simulink library "Index2DbTableBtc"  (R2022b)
settings: Solver=VariableStepAuto  StartTime=0.0  StopTime=10.0  RelTol=1e-3
undefined symbols (not defined in the file or in its folder): Config, Row
libraries: TuneVar x3, TOP x2, HandyTextFile x1
settings Model: Creator=kl13806  LastModifiedBy=kl13806
settings SolverCC: AlgebraicLoopSolver=TrustRegion
settings DebuggingCC: UnconnectedInputMsg=warning  UnconnectedOutputMsg=warning  UnconnectedLineMsg=warning  SFMachineParentedDataDiag=warning
settings ModelReferenceCC: EnableRefExpFcnMdlSchedulingChecks=on
settings RTWCC: DLArmComputeVersion=19.05

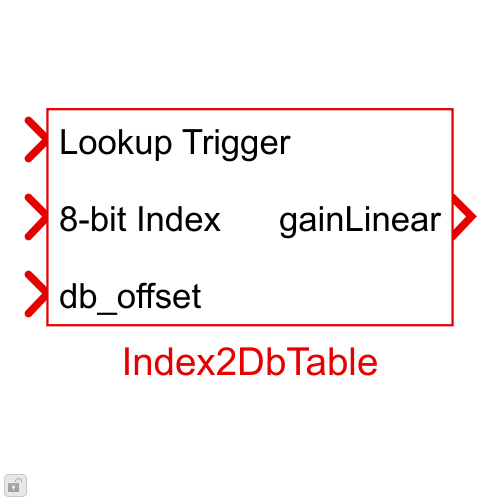
[thumbnail: Simulink's stored preview of the top-level diagram]
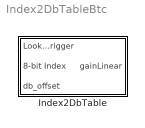
== system Index2DbTableBtc ==
  Index2DbTable : Subsystem  mask(Blocklib Index2DbTable){Config=Config}
      mask prompts: Config "Index2DbTableConfig"
      mask help: This block contains overlay tuning data for an index-to-dB lookup table. Provide the maximum number of points in the table as a build-time variable. The TuneVar is variable size, but must define at least two points (i.e. two rows, or four values).
      mask init:
      | blkh=gcbh;
      | Config=BTConfig.Assert(blkh,Config);
      | 
      | Config.Validate();
      mask Help:
      | This block contains overlay tuning data which defines an index-to-dB lookup table.
      | Each row of the tuning data contains an index and a dB value.
      | 
      | Tuning data
      | ---------------
      |    tune index: normalized value between 0 and 1
      |    tune value: dB value such as 0 (aka linear "1") or -100 (aka "very quiet")
      | 
      | Inports
      | ----------
      |    trigger: function call trigger that invokes the lookup from inport index to output dB
      |    index: an 8-bit integer index between [0:255] corresponding to the tuning index range [0:1]
      | 
      | Outport
      | -----------
      |    The resulting dB value looked up in the tuned table by using the inbound index

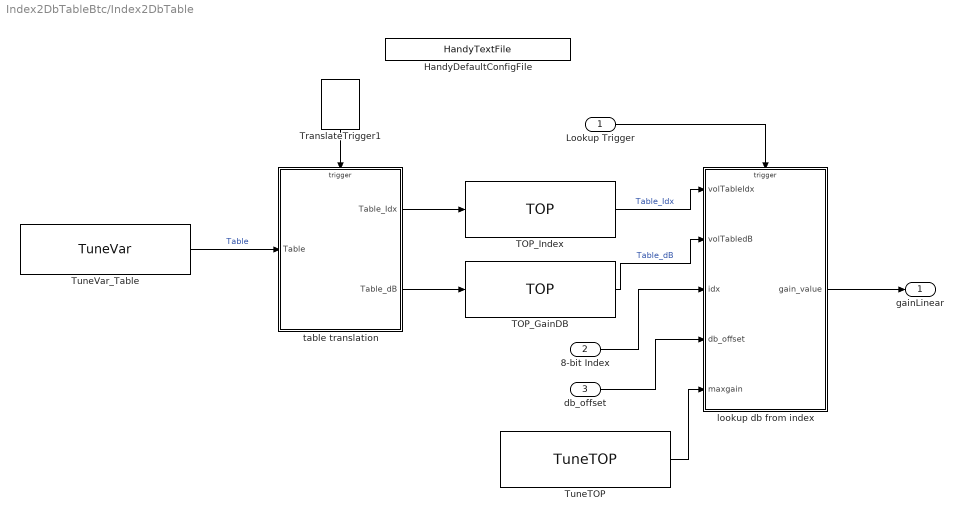
== system Index2DbTableBtc/Index2DbTable ==
  Lookup Trigger : Inport
  8-bit Index : Inport  Port=2
  db_offset : Inport  Port=3
  HandyDefaultConfigFile : HandyTextFile/HandyTextFile  TemplateSource=Config  FileSuffix=Init  OpenDialogOnLoad=off  UseThisBlockName=off  AddGrandParentNamePrefix=off  TheDefaultText=|  ShowInLibBrowser=on
      | % $(FILENAME) Setup model parameters for each "Init" callback (e.g. update diagram)
      | sample_rate_in_hertz = 44100;
      | frame_size = 32;
      | sysin_channel_count = 2;
      settings: SourceProductName=Bose Talaria
  TOP_GainDB : TOP/TOP  TriggerInit=[635 177 785 233]  TopName=Table_dB  DataType=Inherit: Same as input  BankNumber=Config.BankNumber  PreOverlay=false  PostOverlay=false  Role=Automatic
      settings: SourceProductName=Bose Talaria
  TOP_Index : TOP/TOP  TriggerInit=[635 97 785 153]  TopName=Table_Idx  DataType=Inherit: Same as input  BankNumber=Config.BankNumber  PreOverlay=false  PostOverlay=false  Role=Automatic
      settings: SourceProductName=Bose Talaria
  TranslateTrigger1 : TuneVar/TranslateTrigger  TriggerInit=[491 -5 529 45]
      settings: SourceProductName=Bose Talaria
  TuneTOP : TuneVar/TuneTOP  Description=Variable limits the maximum *dB offset* which will be applied to the gain as part of table lookup. It does *not* directly impact the maximum gain applied, only the maximum dB offset.  TriggerInit=[670 347 840 403]  TopName=maxgain  TuneName=maxgain  DataType=single  TunabilityNumber=1  MinValue=[]  MaxValue=[]  BankNumber=0  PreOverlay=false  PostOverlay=false  UseSameName=on  MaskValue=Config.DefaultMaxDbOffset
      settings: SourceProductName=Bose Talaria
  TuneVar_Table : TuneVar/TuneVar  Description=|  TuneName=Table  SpecifyMaxSize=on  VariableDim=1 (Row)  MaxSize=[Config.MaximumTablePoints 2]  TunabilityNumber=2  MinValue=[0;-100]  MaxValue=[1;0]  TriggerInit=[190 140 360 190]  MaskValue=Config.DefaultTable
      | <HTML>Gain table maps index to gain.
      | The index values are <FONT color="red">normalized</Font> floats between 0 and 1 while the gains are in dB (i.e. 0 implies no attenuation).
      | </html>
      settings: SourceProductName=Bose Talaria
  lookup db from index : MATLAB Function  TreatAsAtomicUnit=on
  table translation : MATLAB Function  TreatAsAtomicUnit=on
  gainLinear : Outport  VectorParamsAs1DForOutWhenUnconnected=off
  wires:
  TuneTOP/1 -> lookup db from index/5(maxgain)
  db_offset/1 -> lookup db from index/4(db_offset)
  TuneVar_Table/1 -> table translation/1(Table)  "Table"
  TranslateTrigger1/1 -> table translation/Trigger
  table translation/1(Table_Idx) -> TOP_Index/1
  TOP_GainDB/1 -> lookup db from index/2(volTabledB)  "Table_dB"
  table translation/2(Table_dB) -> TOP_GainDB/1
  TOP_Index/1 -> lookup db from index/1(volTableIdx)  "Table_Idx"
  lookup db from index/1(gain_value) -> gainLinear/1
  Lookup Trigger/1 -> lookup db from index/Trigger
  8-bit Index/1 -> lookup db from index/3(idx)

== matlab function Index2DbTableBtc/Index2DbTable/lookup db from index ==
  data: volTableIdx input; volTabledB input; idx input; gain_value output; db_offset input int32; maxgain input
  events: trigger input FUNCTION_CALL_EVENT
function gain_value = LookupTheDB(volTableIdx, volTabledB, idx, db_offset, maxgain)
%#codegen
%
% Lookup volume table 
% Output Gain vlue from table
%

j = uint8(1);
gain_value = single(0.0);
interpolated_gain_dB=single(0.0);
interpolated_gain_dB_with_offset=single(0.0);

% workaround to type problem
idx = cast(idx, class(volTableIdx(end)));

%  bounds checking for vol - clip to max idx
if (idx > volTableIdx(end))
    idx = volTableIdx(end);
end
%  bounds checking for gain offset(No Boost) - clip to max offset level
if (db_offset > int32(maxgain))
    db_offset = int32(maxgain);
end
if (db_offset < int32(-10.0))
    db_offset = int32(-10.0);
end

% search through volume table to find index closest to vol
while (j <= numel(volTableIdx))
    if (idx <= volTableIdx(j))
        if (j <= 1)  % first indexed value is linearly interpolated to zero
            if (volTableIdx(j))
                percent = single(idx) / single(volTableIdx(j));
            else
                percent = single(1);
            end
            gain_value = percent * 10 ^ ( (volTabledB(j)+ single(db_offset)) / 20);
        else         % other values are interpolated in db space
            lastIdx = volTableIdx(j-1);
            percent = single(idx - lastIdx) / single(volTableIdx(j) - lastIdx);
            interpolated_gain_dB = (percent * (volTabledB(j) - volTabledB(j-1) ) ) + volTabledB(j-1);
            interpolated_gain_dB_with_offset= interpolated_gain_dB + single(db_offset); 
            gain_value = 10 ^ ( (interpolated_gain_dB_with_offset) / 20);            
        end
        break;
    else
        j = j + 1;
    end
end

== matlab function Index2DbTableBtc/Index2DbTable/table translation ==
  data: Table_Idx output; Table_dB output; Table input
  events: trigger input FUNCTION_CALL_EVENT
function [Table_Idx,Table_dB] = fcn(Table)
%#codegen
%
% Demux table matrix into one dimesional value and index vectors
%
%
% Set up the size and datatype of our TOP outputs:
maxTableSize = numel(Table.Value) / 2;
idxType = 'uint8';
idxStorageType = 'uint32';
dbType = 'single';
Table_Idx = zeros(1,maxTableSize,idxStorageType);
Table_dB = zeros(1,maxTableSize,dbType);

% separate the pairs into their index and value components
givenPairs = Table.Size(1);
indexes = Table.Value(1:givenPairs,1);
values = Table.Value(1:givenPairs,2);

% then sort and ignore duplicates
[cleanIdx,map] = unique(indexes);

% Validate input sizes
numPairs = numel(map);
argName='Table';

% Validate: enough data?
if (numPairs < 2)
    TranslateError('%s must have at least 2 index pairs. Encounted value with only %f pairs\n', argName, numPairs);
end

% Validate: Highest index still below 1.0?
if (cleanIdx(end) > 1)
    TranslateError('%s out of range table index %f encountered. Index must be between 0 and 1.\n',argName,cleanIdx(end));
end

% fill in the table buffer with provided pairs
for i=1:numPairs
    Table_Idx(i) = intmax(idxType) * cleanIdx(i);
    Table_dB(i) = values(map(i));
end
% fill the rest of the table buffer with the last entry
for j=numel(map)+1:maxTableSize
    Table_Idx(j) = Table_Idx(numPairs);
    Table_dB(j) =  Table_dB(numPairs);
end

end
